simulink model "ROBOT_HW"  (R2015b)
settings: Solver=ode45  StartTime=0.0  StopTime=20  RelTol=1e-3
undefined symbols (not defined in the file): g, i1, i2, l1, l2, m1, m2
libraries: simulink x4
settings Model: Creator=ihong-gyu  LastModifiedBy=ihong-gyu

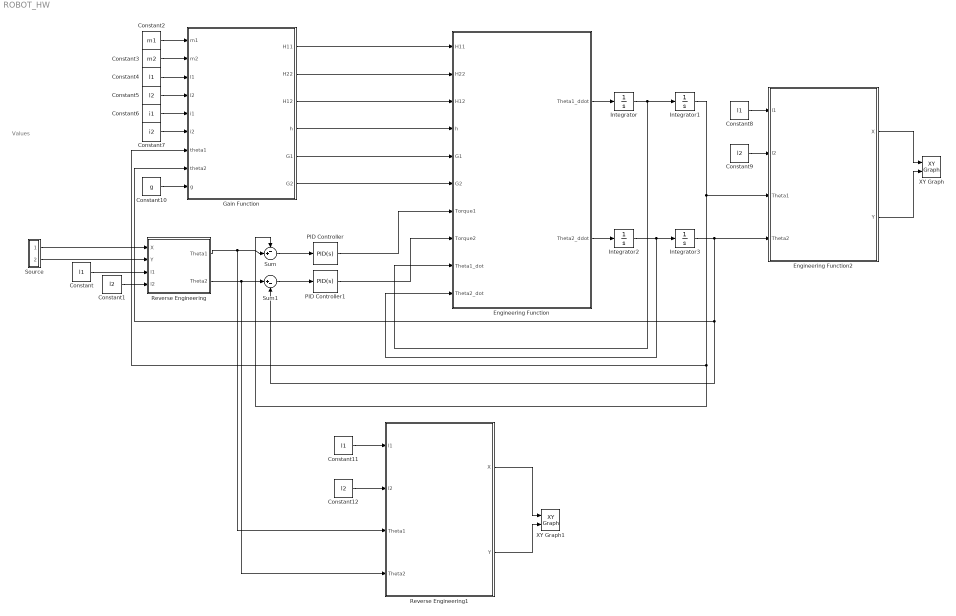
== system ROBOT_HW ==
  note: Values
  Constant{,4,8,11} (4 alike) : Constant  Value=l1
  Constant{1,5,9,12} (4 alike) : Constant  Value=l2
  Constant10 : Constant  Value=g
  Constant2 : Constant  Value=m1
  Constant3 : Constant  Value=m2
  Constant6 : Constant  Value=i1
  Constant7 : Constant  Value=i2
  Engineering Function : MATLAB Function  TreatAsAtomicUnit=on
  Engineering Function2 : MATLAB Function  TreatAsAtomicUnit=on
  Gain Function : MATLAB Function  TreatAsAtomicUnit=on
  Integrator : Integrator
  Integrator1 : Integrator  InitialCondition=-0.35
  Integrator2 : Integrator
  Integrator3 : Integrator  InitialCondition=1.7
  PID Controller : simulink/Continuous/PID Controller  Controller=PID  TimeDomain=Continuous-time  SampleTime=-1  IntegratorMethod=Forward Euler  FilterMethod=Forward Euler  Form=Parallel  UseFilter=on  ControllerParametersSource=internal  P=200  I=170  D=180  N=500  InitialConditionSource=internal  InitialConditionForIntegrator=0  InitialConditionForFilter=0  ExternalReset=none  LimitOutput=off  UpperSaturationLimit=inf  LowerSaturationLimit=-inf  LinearizeAsGain=on  AntiWindupMode=none  Kb=1  TrackingMode=off  Kt=1  PParamMin=[]  PParamMax=[]  IParamMin=[]  IParamMax=[]  DParamMin=[]  DParamMax=[]  NParamMin=[]  NParamMax=[]  KbParamMin=[]  KbParamMax=[]  KtParamMin=[]  KtParamMax=[]  POutMin=[]  POutMax=[]  IOutMin=[]  IOutMax=[]  DOutMin=[]  DOutMax=[]  NOutMin=[]  NOutMax=[]  KbOutMin=[]  KbOutMax=[]  KtOutMin=[]  KtOutMax=[]  IntegratorOutMin=[]  IntegratorOutMax=[]  FilterOutMin=[]  FilterOutMax=[]  SumOutMin=[]  SumOutMax=[]  SumI1OutMin=[]  SumI1OutMax=[]  SumI2OutMin=[]  SumI2OutMax=[]  SumI3OutMin=[]  SumI3OutMax=[]  SumDOutMin=[]  SumDOutMax=[]  SaturationOutMin=[]  SaturationOutMax=[]  IntegratorContinuousStateAttributes=''  IntegratorStateMustResolveToSignalObject=off  IntegratorRTWStateStorageClass=Auto  FilterContinuousStateAttributes=''  FilterStateMustResolveToSignalObject=off  FilterRTWStateStorageClass=Auto  DifferentiatorICPrevScaledInput=0  DifferentiatorOutMin=[]  DifferentiatorOutMax=[]
  PID Controller1 : simulink/Continuous/PID Controller  Controller=PID  TimeDomain=Continuous-time  SampleTime=-1  IntegratorMethod=Forward Euler  FilterMethod=Forward Euler  Form=Parallel  UseFilter=on  ControllerParametersSource=internal  P=250  I=170  D=180  N=500  InitialConditionSource=internal  InitialConditionForIntegrator=0  InitialConditionForFilter=0  ExternalReset=none  LimitOutput=off  UpperSaturationLimit=inf  LowerSaturationLimit=-inf  LinearizeAsGain=on  AntiWindupMode=none  Kb=1  TrackingMode=off  Kt=1  PParamMin=[]  PParamMax=[]  IParamMin=[]  IParamMax=[]  DParamMin=[]  DParamMax=[]  NParamMin=[]  NParamMax=[]  KbParamMin=[]  KbParamMax=[]  KtParamMin=[]  KtParamMax=[]  POutMin=[]  POutMax=[]  IOutMin=[]  IOutMax=[]  DOutMin=[]  DOutMax=[]  NOutMin=[]  NOutMax=[]  KbOutMin=[]  KbOutMax=[]  KtOutMin=[]  KtOutMax=[]  IntegratorOutMin=[]  IntegratorOutMax=[]  FilterOutMin=[]  FilterOutMax=[]  SumOutMin=[]  SumOutMax=[]  SumI1OutMin=[]  SumI1OutMax=[]  SumI2OutMin=[]  SumI2OutMax=[]  SumI3OutMin=[]  SumI3OutMax=[]  SumDOutMin=[]  SumDOutMax=[]  SaturationOutMin=[]  SaturationOutMax=[]  IntegratorContinuousStateAttributes=''  IntegratorStateMustResolveToSignalObject=off  IntegratorRTWStateStorageClass=Auto  FilterContinuousStateAttributes=''  FilterStateMustResolveToSignalObject=off  FilterRTWStateStorageClass=Auto  DifferentiatorICPrevScaledInput=0  DifferentiatorOutMin=[]  DifferentiatorOutMax=[]
  Reverse Engineering : MATLAB Function  TreatAsAtomicUnit=on
  Reverse Engineering1 : MATLAB Function  TreatAsAtomicUnit=on
  Source : Subsystem
  Sum : Sum  Inputs=-+|
  Sum1 : Sum  Inputs=|+-
  XY Graph : simulink/Sinks/XY Graph  xmin=-20  xmax=30  ymin=-20  ymax=30  st=-1
  XY Graph1 : simulink/Sinks/XY Graph  xmin=-20  xmax=30  ymin=-20  ymax=30  st=-1
  wires:
  Source/1(X) -> Reverse Engineering/1(X)
  Source/2(Y) -> Reverse Engineering/2(Y)
  Reverse Engineering/2(Theta2) -> Reverse Engineering1/4(Theta2), Sum1/1
  Constant/1 -> Reverse Engineering/3(l1)
  Constant1/1 -> Reverse Engineering/4(l2)
  Sum1/1 -> PID Controller1/1
  Sum/1 -> PID Controller/1
  Constant2/1 -> Gain Function/1(m1)
  Constant3/1 -> Gain Function/2(m2)
  Constant4/1 -> Gain Function/3(l1)
  Constant5/1 -> Gain Function/4(l2)
  Constant6/1 -> Gain Function/5(i1)
  Constant7/1 -> Gain Function/6(i2)
  Constant10/1 -> Gain Function/9(g)
  PID Controller/1 -> Engineering Function/7(Torque1)
  PID Controller1/1 -> Engineering Function/8(Torque2)
  Integrator/1 -> Engineering Function/9(Theta1_dot), Integrator1/1
  Integrator2/1 -> Engineering Function/10(Theta2_dot), Integrator3/1
  Gain Function/1(H11) -> Engineering Function/1(H11)
  Gain Function/2(H22) -> Engineering Function/2(H22)
  Gain Function/3(H12) -> Engineering Function/3(H12)
  Gain Function/4(h) -> Engineering Function/4(h)
  Gain Function/5(G1) -> Engineering Function/5(G1)
  Gain Function/6(G2) -> Engineering Function/6(G2)
  Integrator1/1 -> Sum/1, Gain Function/7(theta1), Engineering Function2/3(Theta1)
  Integrator3/1 -> Sum1/2, Gain Function/8(theta2), Engineering Function2/4(Theta2)
  Constant8/1 -> Engineering Function2/1(l1)
  Constant9/1 -> Engineering Function2/2(l2)
  Engineering Function/1(Theta1_ddot) -> Integrator/1
  Engineering Function/2(Theta2_ddot) -> Integrator2/1
  Engineering Function2/1(X) -> XY Graph/1
  Engineering Function2/2(Y) -> XY Graph/2
  Reverse Engineering/1(Theta1) -> Reverse Engineering1/3(Theta1), Sum/2
  Constant11/1 -> Reverse Engineering1/1(l1)
  Constant12/1 -> Reverse Engineering1/2(l2)
  Reverse Engineering1/1(X) -> XY Graph1/1
  Reverse Engineering1/2(Y) -> XY Graph1/2

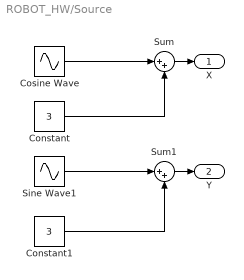
== system ROBOT_HW/Source ==
  Constant : Constant  Value=3
  Constant1 : Constant  Value=3
  Cosine Wave : Sin  Amplitude=3  Phase=pi/2  SampleTime=0
  Sine Wave1 : Sin  Amplitude=3  SampleTime=0
  Sum : Sum  Inputs=|++
  Sum1 : Sum  Inputs=|++
  X : Outport
  Y : Outport  Port=2
  wires:
  Constant/1 -> Sum/2
  Sine Wave1/1 -> Sum1/1
  Constant1/1 -> Sum1/2
  Sum/1 -> X/1
  Sum1/1 -> Y/1
  Cosine Wave/1 -> Sum/1

== matlab function ROBOT_HW/Gain Function ==
  data: m1 input; H11 output; m2 input; H22 output; l1 input; l2 input; i1 input; i2 input; theta1 input; theta2 input; g input; H12 output; h output; G1 output; G2 output
function [H11,H22,H12,h,G1,G2] = fcn(m1,m2,l1,l2,i1,i2,theta1,theta2,g)
%#codegen

H11 = m1*((l1/2)^2) + i1 + m2*((l1^2)+((l2/2)^2)+l1*l2*cos(theta2))+ i2;
H22 = m2*((l2/2)^2) + i2;
H12 = m2*l1*l2/2*cos(theta2)+m2*((l2/2)^2)+i2;
h = m2*l1*l2/2*sin(theta2);
G1 = m1*(l1/2)*g*cos(theta1) + m2*g*((l2/2)*cos(theta1+theta2)+l1*cos(theta1));
G2 = m2*(l2/2)*g*cos(theta1+theta2);

== matlab function ROBOT_HW/Reverse Engineering ==
  data: X input; Theta1 output; Y input; Theta2 output; l1 input; l2 input
function [Theta1,Theta2] = fcn(X,Y,l1,l2)
%#codegen

Theta1 = atan(Y/X) - acos((X^2+Y^2+l1^2-l2^2)/(2*sqrt(X^2+Y^2)*l1));
Theta2 = acos((X^2+Y^2-l1^2-l2^2)/(2*l1*l2));

== matlab function ROBOT_HW/Engineering Function ==
  data: H11 input; H22 input; H12 input; h input; G1 input; G2 input; Torque1 input; Torque2 input; Theta1_ddot output; Theta1_dot input; Theta2_dot input; Theta2_ddot output
function [Theta1_ddot,Theta2_ddot] = fcn(H11,H22,H12,h,G1,G2,Torque1,Torque2,Theta1_dot,Theta2_dot)
%#codegen

Theta1_ddot = (1/(H11*H22-H12^2))*(H22*(Torque1 + h*(Theta2_dot^2) + 2*h*Theta1_dot*Theta2_dot - G1) - H12*(Torque2 - h*(Theta1_dot^2) - G2));
Theta2_ddot = (1/(H11*H22-H12^2))*(-H12*(Torque1 + h*(Theta2_dot^2) + 2*h*Theta1_dot*Theta2_dot - G1) + H11*(Torque2 - h*(Theta1_dot^2) - G2));

== matlab function ROBOT_HW/Engineering Function2 ==
  data: l1 input; l2 input; Theta1 input; X output; Theta2 input; Y output
function [X,Y] = fcn(l1,l2,Theta1,Theta2)
%#codegen

X = l1*cos(Theta1)+l2*cos(Theta1+Theta2);
Y = l1*sin(Theta1)+l2*sin(Theta1+Theta2);

== matlab function ROBOT_HW/Reverse Engineering1 ==
  data: l1 input; l2 input; Theta1 input; X output; Theta2 input; Y output
function [X,Y] = fcn(l1,l2,Theta1,Theta2)
%#codegen

X = l1*cos(Theta1)+l2*cos(Theta1+Theta2);
Y = l1*sin(Theta1)+l2*sin(Theta1+Theta2);
